simulink model "SCARA"  (R2018a)
settings: Solver=VariableStepAuto  StartTime=0.0  StopTime=10.0  RelTol=1e-3
model workspace: external: MATLAB File C:\Users\1511 MXTI\Desktop\CEFET\ROBÓTICA\SCARA 4\SCARA4_DataFile1.m (data not in the file)
undefined symbols (not defined in the file or in its folder): smiData, X, Y, Z
libraries: sm_lib x20, nesl_utility x9
(part 2 of 2)

== matlab function SCARA/M ==
  data: Izz1 input; M output; Izz2 input; Izz3 input; L1 input; L2 input; m1 input; m2 input; m3 input; q2 input; q4 input; xG1 input; xG2 input; xG3 input; yG1 input; yG2 input; yG3 input
function M = M(Izz1,Izz2,Izz3,L1,L2,m1,m2,m3,q2,q4,xG1,xG2,xG3,yG1,yG2,yG3)
%#codegen

%    This function was generated by the Symbolic Math Toolbox version 8.6.
%    30-Apr-2021 16:43:47

t2 = cos(q2);
t3 = cos(q4);
t4 = sin(q2);
t5 = sin(q4);
t6 = q2+q4;
t7 = L1.^2;
t8 = L2.^2;
t9 = xG2.^2;
t10 = xG3.^2;
t11 = yG2.^2;
t12 = yG3.^2;
t17 = L2.*m2.*xG2.*2.0;
t13 = cos(t6);
t14 = sin(t6);
t15 = m2.*t8;
t16 = m3.*t8;
t18 = m2.*t9;
t19 = m3.*t10;
t20 = m2.*t11;
t21 = m3.*t12;
t22 = L1.*L2.*m2.*t2;
t23 = L1.*L2.*m3.*t2;
t24 = L1.*m2.*t2.*xG2;
t25 = L2.*m3.*t3.*xG3;
t26 = L1.*m2.*t4.*yG2;
t27 = L2.*m3.*t5.*yG3;
t28 = t25.*2.0;
t29 = t27.*2.0;
t30 = L1.*m3.*t13.*xG3;
t31 = L1.*m3.*t14.*yG3;
t32 = -t26;
t33 = -t27;
t34 = -t29;
t35 = -t31;
t36 = Izz3+t19+t21+t25+t33;
t37 = t30+t35+t36;
t38 = Izz2+Izz3+t15+t16+t17+t18+t19+t20+t21+t22+t23+t24+t28+t30+t32+t34+t35;
M = reshape([Izz1+Izz2+Izz3+t15+t16+t17+t18+t19+t20+t21+t22.*2.0+t23.*2.0+t24.*2.0-t26.*2.0+t28+t30.*2.0-t31.*2.0+t34+m1.*t7+m2.*t7+m3.*t7+m1.*xG1.^2+m1.*yG1.^2+L1.*m1.*xG1.*2.0,t38,0.0,t37,t38,Izz2+Izz3+t15+t16+t17+t18+t19+t20+t21+t28+t34,0.0,t36,0.0,0.0,m3,0.0,t37,t36,0.0,Izz3+t19+t21],[4,4]);

== matlab function SCARA/MATLAB Function4 ==
  data: Ts input; qd input; dqd input; d2qd input; qs input; dqs input; M input; Tc output; H input; G input; D input; Kp output; Kd output
function [Tc,Kp,Kd] = Controlador(Ts,qd, dqd, d2qd, qs, dqs, M, H, G, D)

e= qd - qs;
de = dqd - dqs;

% Ts = 4/Zeta*Wn
% Para um sistema criticamente amortecido Zeta = 1
Zeta=1;
Wn= 5/Ts;

%Para equação linear "d2e+Kd*de+Kp*e=0"
Kd=2*Zeta*Wn;
Kp=Wn^2;

MKp = [Kp 0 0 0;0 Kp 0 0;0 0 Kp 0; 0 0 0 Kp];
MKd = [Kd 0 0 0;0 Kd 0 0;0 0 Kd 0; 0 0 0 Kd];

Tc = M*(d2qd + MKd*de + MKp*e) + H + G + D;
end

== matlab function SCARA/MATLAB Function5 ==
  data: M input; d2qs output; Tc input; H input; G input; D input
function d2qs = Planta(M, Tc, H, G, D)

d2qs = inv(M)*(Tc - H - G - D);
end

== matlab function SCARA/MATLAB Function6 ==
  data: horario output; teta output; x output; t input; y output; tf input; z output; dx output; dy output; dz output; ddx output; ddy output; ddz output; alfa output; dalfa output; d2alfa output; R0 input; Rf input; teta0 input; tetaf input; alfa0 input; alfaf input; h0 input; hf input
function [horario,teta,x,y,z,dx,dy,dz,ddx,ddy,ddz,alfa,dalfa,d2alfa] = Trajetoria_da_Ferramenta(t,tf,R0,Rf,teta0,tetaf,alfa0,alfaf,h0,hf)

%% Escolhendo o sentido baseado na menor distância

tetaf1 = tetaf
horario=0;
% if (abs(tetaf)-abs(teta0)) >= (1.98*pi)
%     tetaf = tetaf-(2*pi);
% end
% 
% if (abs(teta0)-abs(tetaf))>=(1.98*pi)
%     teta0=teta0-(2*pi)
% end
    
if tetaf1 >= teta0
    if tetaf1 > (teta0 + pi)
        tetaf = tetaf1-(2*pi);
        horario=1;
    end
else %tetaf1 < teta0
    horario=1;
    if (teta0-pi > tetaf1)
        tetaf = tetaf1+(2*pi);
        horario=0;
    end
end

 

aux = [1 0 0 0;0 1 0 0;1 tf tf^2 tf^3;0 1 2*tf 3*tf^2];
 
a = inv(aux)*[teta0;0;tetaf;0];
teta = a(1) + a(2)*t + a(3)*t^2 + a(4)*t^3;
dteta = a(2) + 2*a(3)*t + 3*a(4)*t^2;
d2teta = 2*a(3) + 6*a(4)*t;

 

b = inv(aux)*[R0;0;Rf;0];
R = b(1) + b(2)*t + b(3)*t^2 + b(4)*t^3;
dR = b(2) + 2*b(3)*t + 3*b(4)*t^2;
d2R = 2*b(3) + 6*b(4)*t;

 

x = R*cos(teta);
dx = -R*sin(teta)*dteta;
ddx = -R*cos(teta)*dteta^2 -R*sin(teta)*d2teta;

 

y = R*sin(teta);
dy = R*cos(teta)*dteta;
ddy = -R*sin(teta)*dteta^2 + R*cos(teta)*d2teta;


c = inv(aux)*[alfa0;0;alfaf;0];
alfa = c(1) + c(2)*t + c(3)*t^2 + c(4)*t^3;
dalfa = c(2) + 2*c(3)*t + 3*c(4)*t^2;
d2alfa = 2*c(3) + 6*c(4)*t;


 
d = inv(aux)*[h0;0;hf;0];
z = d(1) + d(2)*t + d(3)*t^2 + d(4)*t^3;
dz = d(2) + 2*d(3)*t + 3*d(4)*t^2;
ddz = 2*d(3) + 6*d(4)*t;
% 
% z=0
% dz=0;
% ddz=0;

end

== matlab function SCARA/MATLAB Function7 ==
  data: horario input; phiAnterior input; phi output; q1 output; x input; q2 output; y input; z input; dx input; dy input; dz input; d2x input; d2y input; d2z input; L0 input; L1 input; L2 input; e1 input; q3 output; alfa input; q4 output; dq1d output; dq2d output; dq3d output; dq4d output; d2q1d output; d2q2d output; d2q3d output; d2q4d output; dalfa input; ddalfa input
function [phi, q1 ,q2, q3, q4, dq1d, dq2d, dq3d, dq4d, d2q1d, d2q2d, d2q3d, d2q4d] = CinInvAng(horario,phiAnterior,x,y,z,dx,dy,dz,d2x,d2y,d2z,L0,L1,L2,e1,alfa,dalfa,ddalfa)

phiAnterior=1;
d = sqrt(x^2 + y^2);
beta = acos((L1^2 + L2^2 - d^2)/(2*L1*L2));
alfa2 = asin(L2*sin(beta)/d);
gama = asin(L1*sin(beta)/d);

%% POSIÇÃO DAS JUNTAS
     
%PRIMEIRO E SEGUNDO QUADRANTE
if y>=0
    if horario == 0             % SENTIDO ANTI-HORÁRIO
        phi = atan2(y,x);
        q1 = phi - alfa2;
    else                        % SENTIDO HORÁRIO
        phi = atan2(y,x);
        q1 = phi+alfa2;
    end
else                            % TERCEIRO E QUARTO QUADRANTE
    if horario == 0             % SENTIDO ANTI-HORÁRIO
        phi = atan2(y,x);       % PHI NESTES QUADRANTE É NEGATIVO USANDO ATAN2
        q1 =(2*pi)-alfa2+phi;
    else                        % SENTIDO HORÁRIO
        phi = atan2(y,x);       % PHI NESTES QUADRANTE É NEGATIVO USANDO ATAN2
        q1 = phi+alfa2
    end
end

if horario == 0                 % SENTIDO ANTI-HORÁRIO
    q2 = (pi - beta);
else                            % SENTIDO HORÁRIO
    q2 = -(pi - beta);
end

q3 = z-L0-e1;
q4 = alfa - q1 - q2;

%% VELOCIDADE DAS JUNTAS

VL = [dx;dy;dz];
JL = [- L2*sin(q1 + q2) - L1*sin(q1), -L2*sin(q1 + q2), 0;L2*cos(q1 + q2) + L1*cos(q1),  L2*cos(q1 + q2), 0;0, 0, 1];
dq = inv(JL)*VL;
dq1d = dq(1);
dq2d = dq(2);
dq3d = dq(3);
dq4d = dalfa - dq1d - dq2d;


%% ACELERAÇÃO DAS JUNTAS

aL = [d2x;d2y;d2z];
JL = [- L2*sin(q1 + q2) - L1*sin(q1), -L2*sin(q1 + q2), 0;L2*cos(q1 + q2) + L1*cos(q1),  L2*cos(q1 + q2), 0;0, 0, 1];
dJL = [- dq1d*(L2*cos(q1 + q2) + L1*cos(q1)) - L2*dq2d*cos(q1 + q2), -L2*cos(q1 + q2)*(dq1d + dq2d), 0;- dq1d*(L2*sin(q1 + q2) + L1*sin(q1)) - L2*dq2d*sin(q1 + q2), -L2*sin(q1 + q2)*(dq1d + dq2d), 0;0, 0, 0];
d2qd = inv(JL)*aL - (dJL*[q1;q2;q3]);

d2q1d = d2qd(1);
d2q2d = d2qd(2);
d2q3d = d2qd(3);
d2q4d = ddalfa - d2q1d - d2q2d;

end

== matlab function SCARA/TRAMENTO DAS ENTRADAS/MATLAB Function8 ==
  data: t input; tf input; R0 input; Rf input; teta0 input; tetaf input; alfa0 input; alfaf input; t output; tf output; R0 output; Rf output; teta0 output; tetaf output; alfa0 output; alfaf output; h0 output; h0 input; hf input; hf output; L0 input; L1 input; e1 input; L2 input; e2 input; L3 input; L0 output; L1 output; e1 output; L2 output; e2 output; L3 output
function [t,tf,R0,Rf,teta0,tetaf,alfa0,alfaf,h0,hf,L0,L1,e1,L2,e2,L3]   = Tratameto_Das_Entradas(t,tf,R0,Rf,teta0,tetaf,alfa0,alfaf,h0,hf,L0,L1,e1,L2,e2,L3)

%%   h0 representa a Altura inicial da ferramenta
%   h0t representa a Altura inicial da ferramenta tratadas inserindo as
%   condiçoes limites evitando singularidades
if h0 >= (L0+e1-e2)
    h0 =(L0+e1-e2)-0.01;
elseif  hf <= (L0+e1-e2-L3)
    h0=(L0+e1-e2-L3)+0.01;
end

%%   hf representa a Altura final da ferramenta
%   hfaux representa a Altura inicial da ferramenta tratadas inserindo as
%   condiçoes limites evitando singularidades

if hf >= (L0+e1-e2)
    hf =(L0+e1-e2)-0.01;
elseif  hf <= (L0+e1-e2-L3)
    hf=(L0+e1-e2-L3)+0.01;
end

%% Garantindo que o Scara não atinja suas condições limites, 
% Evitando as  singumalridades

if R0 >= (L1+L2)
    R0=0.999*(L1+L2);
elseif R0 <= (L1-L2)
    R0=(L1-L2)+0.4;
end

if Rf >= (L1+L2)
    Rf=0.999*(L1+L2);
elseif Rf <= (L1-L2)
    Rf=(L1-L2)+0.40;
end



end
